simulink model "lab_2_sumlink_module"  (R2023b)
settings: Solver=VariableStepAuto  StartTime=0.0  StopTime=10.0  RelTol=1e-3
settings Model: Creator=ascom  LastModifiedBy=ascom

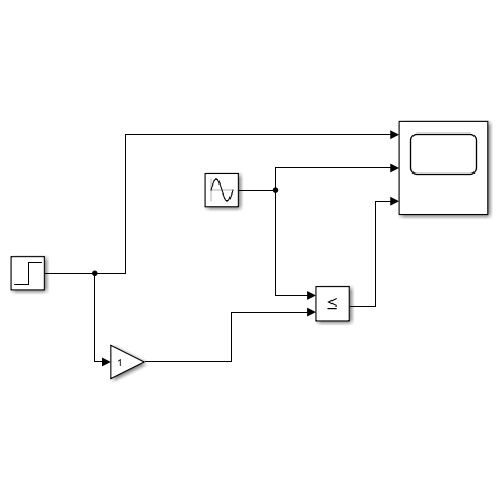
[thumbnail: Simulink's stored preview of the top-level diagram]
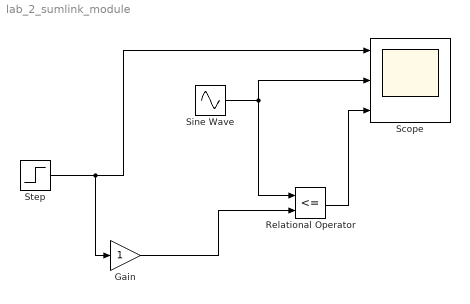
== system lab_2_sumlink_module ==
  Gain : Gain
  Relational Operator : RelationalOperator  Operator=<=  OutDataTypeStr=boolean  RndMeth=Simplest  InputSameDT=off
  Scope : Scope  NumInputPorts=3
  Sine Wave : Sin  SampleTime=0
  Step : Step  Time=2  SampleTime=0
  wires:
  Sine Wave/1 -> Relational Operator/1, Scope/2
  Relational Operator/1 -> Scope/3
  Step/1 -> Gain/1, Scope/1
  Gain/1 -> Relational Operator/2
